simulink model "double_w_haptics"  (Simulink 7.0)
settings: Solver=ode3  StartTime=0.0  StopTime=inf  FixedStep=0.01  RelTol=1e-3
InitFcn:
  | set_global()
values from neighbouring files (symbols this model uses):
  B_I = eye(3)    [Fourbar_init.m]    (also in Update_2bar.m = B_M*     [width^2+depth^2  -R_len*width      -R_len*depth;  ; Update_4bar.m = B_M*     [width^2+depth^2  -R_len*width      -R_len*depth;  )
  B_M = .10    (= 0.1)    [Fourbar_init.m]    (also in Update_2bar.m = str2double(get(obj.Double_base_M, 'String')); Update_4bar.m = str2double(get(obj.R_M, 'String')))
  Bone_I = eye(3)    [Fourbar_init.m]    (also in Update_2bar.m = Bone_M*     [width^2+depth^2  -len*width      -len*depth;   ; Update_4bar.m = Bone_M*     [width^2+depth^2  -len*width      -len*depth;   )
  Bone_M = .50    (= 0.5)    [Fourbar_init.m]    (also in Update_2bar.m = str2double(get(obj.Double_follow_M, 'String')); Update_4bar.m = str2double(get(obj.C_M, 'String')))
  Cd = 9    [Fourbar_init.m]    (also in Update_2bar.m = str2double(get(obj.DAMPER, 'String')); Update_4bar.m = str2double(get(obj.DAMPER, 'String')))
  EE_gain = 14    [Fourbar_init.m]    (also in Update_2bar.m = dia_C / .033; Update_4bar.m = dia_C / .033)
  Gravity = str2num(get(hObject.GRAVITY, 'String'))    [Fourbar.m]    (also in Fourbar_init.m = 0; Update_2bar.m = str2double(get(obj.GRAVITY, 'String')); Update_4bar.m = str2double(get(obj.GRAVITY, 'String')))
  ks = str2num(get(hObject.SPRING, 'String'))    [Fourbar.m]    (also in Fourbar_init.m = 250; Update_2bar.m = str2double(get(obj.SPRING, 'String')); Update_4bar.m = str2double(get(obj.SPRING, 'String')))
libraries: mblibv1 x8, quarc_library x1
settings Model: Creator=colinlea  LastModifiedBy=colinlea  SimulationMode=external  ExtModeTrigDuration=10000
settings SolverCC: PositivePriorityOrder=on
settings ModelReferenceCC: UpdateModelReferenceTargets=IfOutOfDate
settings RTWCC: SystemTargetFile=quarc_windows.tlc  TemplateMakefile=quarc_default_tmf  Description=QuaRC Win32 Target  ProcessScript=quarc_windows_make_rtw_hook
settings STFCustomTargetCC: TargetPreCompLibLocation=C:\DOCUME~1\ALLUSE~1\APPLIC~1\QuaRC\lib\2007b\windows\release  GenFloatMathFcnCalls=ANSI_C  SystemTargetFile=quarc_windows.tlc
settings GRTTargetCC: TargetPreCompLibLocation=C:\DOCUME~1\ALLUSE~1\APPLIC~1\QuaRC\lib\2007b\windows\release  CompOptLevelCompliant=off  MatFileLogging=off  ExtMode=on  ExtModeMexFile=quarc_comm

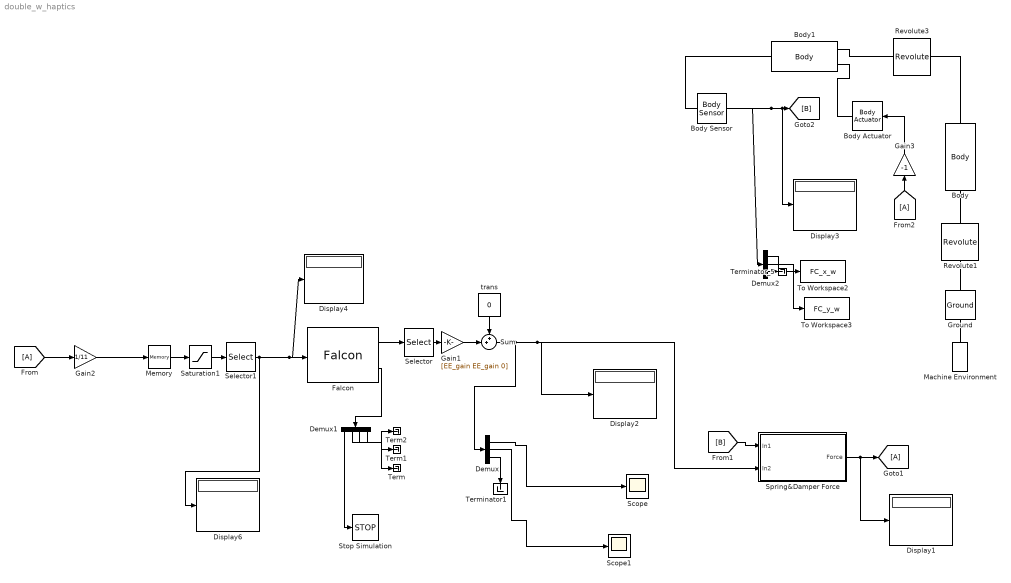
== system double_w_haptics ==
  Body : mblibv1/Bodies/Body  Orientation=up  DialogController=MECH.DynMechDlgSource  PhysicalDomain=mechanical  SubClassName=Unknown  LeftPortType=workingframe  RightPortType=workingframe  LConnTagsString=CS1  RConnTagsString=CS2  DialogClass=MechanicalBodyBlock  Mass=B_M  MassUnits=kg  InertiaUnits=kg*m^2  Inertia=B_I  Shape=Cylinder  ShapeDims=[1 1]  ShapeUnits=m  ShapeUse=false  Density=1  DensityUnits=kg/m^3  DensityUse=false  CG=Left$CG$B_CG_P$World$World$m$[0 0 0]$Euler X-Y-Z$deg$WORLD$false  WorkingFrames=Left$CS1$B_CS1_P$World$World$m$[0 0 0]$Euler X-Y-Z$deg$WORLD$true#Right$CS2$B_CS2_P$World$World$m$[0 0 0]$Euler X-Y-Z$deg$WORLD$true  CGPos=B_CG_P  CGRot=[0 0 0]  CS0Pos=[]  CS0Rot=[]  CS1Pos=B_CS1_P  CS1Rot=[0 0 0]  CS2Pos=B_CS2_P  CS2Rot=[0 0 0]  CS3Pos=[]  CS3Rot=[]  CS4Pos=[]  CS4Rot=[]  CS5Pos=[]  CS5Rot=[]  CS6Pos=[]  CS6Rot=[]  CS7Pos=[]  CS7Rot=[]  CS8Pos=[]  CS8Rot=[]  CS9Pos=[]  CS9Rot=[]  CS10Pos=[]  CS10Rot=[]  CS11Pos=[]  CS11Rot=[]  CS12Pos=[]  CS12Rot=[]  CS13Pos=[]  CS13Rot=[]  CS14Pos=[]  CS14Rot=[]  CS15Pos=[]  CS15Rot=[]  CS16Pos=[]  CS16Rot=[]  CS17Pos=[]  CS17Rot=[]  CS18Pos=[]  CS18Rot=[]  CS19Pos=[]  CS19Rot=[]  CS20Pos=[]  CS20Rot=[]
  Body Actuator : mblibv1/Sensors &  Actuators/Body Actuator  Orientation=left  DialogController=MECH.DynMechDlgSource  SystemSampleTime=-1  PhysicalDomain=Mechanical  PortType=blob  ActuationStyle=Force  AngleUnits=deg  ArcVelocityUnits=deg/s  ArcAccelerationUnits=deg/s^2  CoordPositionUnits=m  VelocityUnits=m/s  AccelerationUnits=m/s^2  ForceUnits=N  TorqueUnits=N*m  ActiveIO=on  Width=3  DialogClass=MechanicalActuatorBlock  ReferenceFrame=Absolute (World)  Angle=off  CoordPosition=on  Force=on  Torque=off
  Body Sensor : mblibv1/Sensors &  Actuators/Body Sensor  DialogController=MECH.DynMechDlgSource  SystemSampleTime=-1  PhysicalDomain=Mechanical  PortType=blob  Muxed=on  Pose=off  Angle=on  AngleUnits=deg  ArcVelocity=off  ArcVelocityUnits=deg/s  ArcAcceleration=off  ArcAccelerationUnits=deg/s^2  CoordPosition=on  CoordPositionUnits=m  Velocity=off  VelocityUnits=m/s  Acceleration=off  AccelerationUnits=m/s^2  Quaternion=on  QuaternionDT=off  QuaternionDDT=off  QuaternionUnits=off  OutputVector=[1]  ActiveIO=on  Width=3  DialogClass=MechanicalSensorBlock  ReferenceFrame=Absolute (World)
  Body1 : mblibv1/Bodies/Body  Orientation=left  DialogController=MECH.DynMechDlgSource  PhysicalDomain=mechanical  SubClassName=Unknown  LeftPortType=workingframe  RightPortType=workingframe  LConnTagsString=CS1|CS4  RConnTagsString=CS3  DialogClass=MechanicalBodyBlock  Mass=Bone_M  MassUnits=kg  InertiaUnits=kg*m^2  Inertia=Bone_I  Shape=Cylinder  ShapeDims=[1 1]  ShapeUnits=m  ShapeUse=false  Density=1  DensityUnits=kg/m^3  DensityUse=false  CG=Left$CG$Bone_CG_P$World$World$m$[0 0 0]$Euler X-Y-Z$deg$WORLD$false  WorkingFrames=Left$CS1$Bone_CS1_P$World$World$m$[0 0 0]$Euler X-Y-Z$deg$WORLD$true#Right$CS2$Bone_CS2_P$World$World$m$[0 0 0]$Euler X-Y-Z$deg$WORLD$false#Right$CS3$[0 0 0]$CS2$CS2$m$[0 0 0]$Euler X-Y-Z$deg$WORLD$true#Left$CS4$[0 0 0]$CS2$CS2$m$[0 0 0]$Euler X-Y-Z$deg$WORLD$true  CGPos=Bone_CG_P  CGRot=[0 0 0]  CS0Pos=[]  CS0Rot=[]  CS1Pos=Bone_CS1_P  CS1Rot=[0 0 0]  CS2Pos=Bone_CS2_P  CS2Rot=[0 0 0]  CS3Pos=[0 0 0]  CS3Rot=[0 0 0]  CS4Pos=[0 0 0]  CS4Rot=[0 0 0]  CS5Pos=[]  CS5Rot=[]  CS6Pos=[]  CS6Rot=[]  CS7Pos=[]  CS7Rot=[]  CS8Pos=[]  CS8Rot=[]  CS9Pos=[]  CS9Rot=[]  CS10Pos=[]  CS10Rot=[]  CS11Pos=[]  CS11Rot=[]  CS12Pos=[]  CS12Rot=[]  CS13Pos=[]  CS13Rot=[]  CS14Pos=[]  CS14Rot=[]  CS15Pos=[]  CS15Rot=[]  CS16Pos=[]  CS16Rot=[]  CS17Pos=[]  CS17Rot=[]  CS18Pos=[]  CS18Rot=[]  CS19Pos=[]  CS19Rot=[]  CS20Pos=[]  CS20Rot=[]
  Demux : Demux  Outputs=3
  Demux1 : Demux  Orientation=down
  Demux2 : Demux  Outputs=3
  Display{1..4,6} (5 alike) : Display
  Falcon : quarc_library/Devices/Third-Party/Novint/Falcon  sample_time=qc_get_step_size  show_calibrate=off
  Gain1 : Gain  Gain=[EE_gain EE_gain 0]  ParameterDataType=sfix(16)  ParameterScaling=2^0  OutDataType=sfix(16)  OutScaling=2^0
  Gain2 : Gain  Gain=1/11  ParameterDataType=sfix(16)  ParameterScaling=2^0  OutDataType=sfix(16)  OutScaling=2^0
  Gain3 : Gain  Orientation=up  Gain=-1  ParameterDataType=sfix(16)  ParameterScaling=2^0  OutDataType=sfix(16)  OutScaling=2^0
  Ground : mblibv1/Bodies/Ground  Orientation=up  DialogController=MECH.DynMechDlgSource  SystemSampleTime=-1  LeftPortType=env  RightPortType=workingframe  PhysicalDomain=Mechanical  DialogClass=GroundBlock  CoordPosition=G_P  CoordPositionUnits=m  StateVectorMgrId=3  MachineId=[4 0]  ShowEnvPort=on
  Machine Environment : mblibv1/Bodies/Machine Environment  Orientation=up  DialogController=MECH.DialogSource  SystemSampleTime=-1  PortType=env  PhysicalDomain=Mechanical  DialogTemplateClass=MECH.MachineEnvironment  SyncWhenCopied=off  Gravity=[0 Gravity 0]  GravityUnits=m/s^2  GravityAsSignal=off  Dimensionality=Auto-detect  AnalysisType=Forward dynamics  LinearAssemblyTolerance=1e-3  LinearAssemblyToleranceUnits=m  AngularAssemblyTolerance=1e-3  AngularAssemblyToleranceUnits=rad  ConstraintSolverType=Stabilizing  ConstraintRelTolerance=1e-4  ConstraintAbsTolerance=1e-4  UseRobustSingularityHandling=off  RedundancyAnalysisToleranceType=Automatically select tolerance  RedundancyAnalysisTolerance=1e-14  StatePerturbationType=Fixed  PerturbationSize=1e-5  VisualizeMachine=on
  Memory : Memory
  Revolute1 : mblibv1/Joints/Revolute  Orientation=up  DialogController=MECH.DynMechDlgSource  PhysicalDomain=mechanical  SubClassName=Unknown  LeftPortType=blob  RightPortType=blob  LConnTagsString=__newl0  RConnTagsString=__newr0  NumSAPorts=0  CutJoint=off  MarkAsCut=off  Primitives=prismatic  PrimitiveProps=R1$WORLD$[0 0 1]$revolute  DialogClass=JointBlock  R1Axis=[0 0 1]
  Revolute3 : mblibv1/Joints/Revolute  Orientation=left  DialogController=MECH.DynMechDlgSource  PhysicalDomain=mechanical  SubClassName=Unknown  LeftPortType=blob  RightPortType=blob  LConnTagsString=__newl0  RConnTagsString=__newr0  NumSAPorts=0  CutJoint=off  MarkAsCut=off  Primitives=prismatic  PrimitiveProps=R1$WORLD$[0 0 1]$revolute  DialogClass=JointBlock  R1Axis=[0 0 1]
  Saturation1 : Saturate  UpperLimit=18  LowerLimit=-18  OutDataType=sfix(16)  OutScaling=2^0
  Scope : Scope
      settings: SaveName=F_x_w2  DataFormat=Array  MaxDataPoints=2000
  Scope1 : Scope
      settings: SaveName=F_y_w2  DataFormat=Array  MaxDataPoints=2000
  Selector : Selector  InputPortWidth=3  IndexOptions=Index vector (dialog)  Indices=[2 3 1]  OutputSizes=1
  Selector1 : Selector  InputPortWidth=3  IndexOptions=Index vector (dialog)  Indices=[3 1 2]  OutputSizes=1
  Spring&Damper Force : Subsystem
  Stop Simulation : Stop
  Sum : Sum  Inputs=++|  OutDataType=sfix(16)  OutScaling=2^0
  Term : Terminator
  Term1 : Terminator
  Term2 : Terminator
  Terminator1 : Terminator
      settings: Orientation=down
  Terminator_5 : Terminator
  To Workspace2 : ToWorkspace  VariableName=FC_x_w  SampleTime=-1  SaveFormat=Array
  To Workspace3 : ToWorkspace  VariableName=FC_y_w  SampleTime=-1  SaveFormat=Array
  trans : Constant  Orientation=down  Value=0  OutDataType=sfix(16)  OutScaling=2^0
  wires:
  [A] -> Gain2/1
  Falcon/1 -> Selector/1
  Selector/1 -> Gain1/1
  Saturation1/1 -> Selector1/1
  Demux/1 -> Scope/1
  Demux/2 -> Scope1/1
  Spring&Damper Force/1(Force) -> [A], Display1/1
  [B] -> Spring&Damper Force/1(In1)
  Body Sensor/1 -> [B], Display3/1, Demux2/1
  [A] -> Gain3/1
  Gain3/1 -> Body Actuator/1
  Demux/3 -> Terminator1/1
  Gain2/1 -> Memory/1
  Memory/1 -> Saturation1/1
  Falcon/2 -> Demux1/1
  Demux1/2 -> Term/1
  Demux1/4 -> Term2/1
  Demux1/3 -> Term1/1
  Selector1/1 -> Display4/1, Falcon/1, Display6/1
  Demux2/1 -> To Workspace2/1
  Demux2/2 -> To Workspace3/1
  Demux1/1 -> Stop Simulation/1
  Demux2/3 -> Terminator_5/1
  Sum/1 -> Display2/1, Spring&Damper Force/2(In2), Demux/1
  Gain1/1 -> Sum/2
  trans/1 -> Sum/1
  connections:
  Machine Environment/RConn1 -- Ground/LConn1
  Body1/LConn1 -- Revolute3/RConn1
  Revolute3/LConn1 -- Body/RConn1
  Body/LConn1 -- Revolute1/RConn1
  Ground/RConn1 -- Revolute1/LConn1
  Body Actuator/RConn1 -- Body1/LConn2
  Body Sensor/LConn1 -- Body1/RConn1

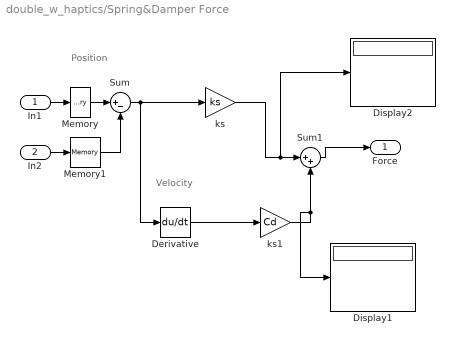
== system double_w_haptics/Spring&Damper Force ==
  note: Position
  note: Velocity
  In1 : Inport
  In2 : Inport  Port=2
  Derivative : Derivative
  Display1 : Display
  Display2 : Display
  Memory : Memory
  Memory1 : Memory
  Sum : Sum  Inputs=|+-  OutDataType=sfix(16)  OutScaling=2^0
  Sum1 : Sum  Inputs=|++  OutDataType=sfix(16)  OutScaling=2^0
  ks : Gain  Gain=ks  ParameterDataType=sfix(16)  ParameterScaling=2^0  OutDataType=sfix(16)  OutScaling=2^0
  ks1 : Gain  Gain=Cd  ParameterDataType=sfix(16)  ParameterScaling=2^0  OutDataType=sfix(16)  OutScaling=2^0
  Force : Outport
  wires:
  Sum1/1 -> Force/1
  Sum/1 -> ks/1, Derivative/1
  ks/1 -> Sum1/1, Display2/1
  Derivative/1 -> ks1/1
  ks1/1 -> Sum1/2, Display1/1
  In1/1 -> Memory/1
  In2/1 -> Memory1/1
  Memory/1 -> Sum/1
  Memory1/1 -> Sum/2
